simulink model "fig9_36"  (Simulink 7.0)
settings: Solver=ode45  StartTime=0.0  StopTime=50.0  RelTol=1e-6
settings Model: Creator=abbas  LastModifiedBy=abbas
settings DataIOCC: SignalLoggingName=sigsOut
settings OptimizationCC: InlineInvariantSignals=on
settings DebuggingCC: SaveWithParameterizedLinksMsg=none  SignalResolutionControl=TryResolveAllWithWarning  SolverPrmCheckMsg=none  MultiTaskDSMMsg=warning  MultiTaskCondExecSysMsg=none  StrictBusMsg=None
settings HardwareCC: TargetUnknown=on
settings RTWCC: IncludeERTFirstTime=on
settings GRTTargetCC: TargetFcnLib=ansi_tfl_tmw.mat  ModelReferenceCompliant=off  CompOptLevelCompliant=off  MatFileLogging=off

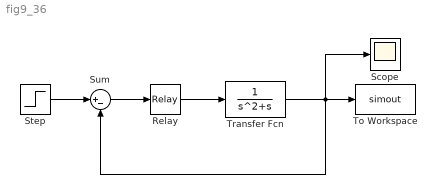
== system fig9_36 ==
  Relay : Relay  OnSwitchValue=0.1  OffSwitchValue=-0.1  OffOutputValue=-1  OutDataType=sfix(16)  OutScaling=2^0
  Scope : Scope
  Step : Step  SampleTime=0
  Sum : Sum  Inputs=|+-  OutDataType=sfix(16)  OutScaling=2^0  SaturateOnIntegerOverflow=on
  To Workspace : ToWorkspace  VariableName=simout  SampleTime=-1  SaveFormat=Array
  Transfer Fcn : TransferFcn  Denominator=[1 1 0]
  wires:
  Relay/1 -> Transfer Fcn/1
  Step/1 -> Sum/1
  Sum/1 -> Relay/1
  Transfer Fcn/1 -> Scope/1, Sum/2, To Workspace/1
